simulink model "gm_uz_pmsm_model_9ph_21b_all_double"  (R2021b)
settings: Solver=FixedStepAuto  StartTime=0.0  StopTime=0.8  RelTol=1e-3
PreLoadFcn:
  | uz_pmsm_model_9ph_init_parameter
undefined symbols (not defined in the file or in its folder): a, b, c, friction_coefficient, inertia, k_i_d, k_i_q, k_p_d, k_p_q, Kpd, L_d, L_o1, L_o2, L_q, L_x1, L_x2, L_y1, L_y2, L_zero, polepair, psi_pm, R_1, static_friction_torque, Tnd, ts
libraries: hdlsllib x90, simulink x32, hdlmdlgenlib x17, dspsigops x7, slpidlib x2, spsAlphaBetaZerotodq0Lib x1, pid_lib x1, spsdq0toAlphaBetaZeroLib x1
(part 4 of 6)

== system gm_uz_pmsm_model_9ph_21b_all_double/uz_pmsm_model_9ph/abc_to_dq/abc_to_dq/_adder_MultiplyAdd12 ==
  in0 : Inport  OutDataTypeStr=fixdt(1, 18, 17)  SampleTime=1e-08
  in1 : Inport  Port=2  OutDataTypeStr=fixdt(1, 25, 12)  SampleTime=1e-08
  in2 : Inport  Port=3  OutDataTypeStr=fixdt(1, 25, 12)  SampleTime=1e-08
  globalSchedule : EnablePort  OutDataTypeStr=boolean
  HwModeRegister : Delay  DelayLength=double(1)  InitialCondition=0
  HwModeRegister1 : Delay  DelayLength=double(1)  InitialCondition=0
  HwModeRegister2 : Delay  DelayLength=double(1)  InitialCondition=0
  PipelineRegister : Delay  DelayLength=double(2)  InitialCondition=0
  _adder_MultiplyAdd : hdlsllib/HDL Operations/Multiply-Add  Function=c+(a.*b)  datatype=fixdt(1, 44, 29)  DoSatur=off  FMA=off
      settings: SourceProductBaseCode=SL
  out0 : Outport  OutDataTypeStr=fixdt(1, 44, 29)  SampleTime=1e-08  InitialOutput=0
  wires:
  PipelineRegister/1 -> out0/1
  in0/1 -> HwModeRegister/1
  in1/1 -> HwModeRegister1/1
  in2/1 -> HwModeRegister2/1
  _adder_MultiplyAdd/1 -> PipelineRegister/1
  HwModeRegister/1 -> _adder_MultiplyAdd/1
  HwModeRegister1/1 -> _adder_MultiplyAdd/2
  HwModeRegister2/1 -> _adder_MultiplyAdd/3

== system gm_uz_pmsm_model_9ph_21b_all_double/uz_pmsm_model_9ph/abc_to_dq/abc_to_dq/_adder_MultiplyAdd13 ==
  in0 : Inport  OutDataTypeStr=fixdt(1, 18, 17)  SampleTime=1e-08
  in1 : Inport  Port=2  OutDataTypeStr=fixdt(1, 25, 12)  SampleTime=1e-08
  in2 : Inport  Port=3  OutDataTypeStr=fixdt(1, 25, 12)  SampleTime=1e-08
  globalSchedule : EnablePort  OutDataTypeStr=boolean
  HwModeRegister : Delay  DelayLength=double(1)  InitialCondition=0
  HwModeRegister1 : Delay  DelayLength=double(1)  InitialCondition=0
  HwModeRegister2 : Delay  DelayLength=double(1)  InitialCondition=0
  PipelineRegister : Delay  DelayLength=double(2)  InitialCondition=0
  _adder_MultiplyAdd : hdlsllib/HDL Operations/Multiply-Add  Function=c+(a.*b)  datatype=fixdt(1, 44, 29)  DoSatur=off  FMA=off
      settings: SourceProductBaseCode=SL
  out0 : Outport  OutDataTypeStr=fixdt(1, 44, 29)  SampleTime=1e-08  InitialOutput=0
  wires:
  PipelineRegister/1 -> out0/1
  in0/1 -> HwModeRegister/1
  in1/1 -> HwModeRegister1/1
  in2/1 -> HwModeRegister2/1
  _adder_MultiplyAdd/1 -> PipelineRegister/1
  HwModeRegister/1 -> _adder_MultiplyAdd/1
  HwModeRegister1/1 -> _adder_MultiplyAdd/2
  HwModeRegister2/1 -> _adder_MultiplyAdd/3

== system gm_uz_pmsm_model_9ph_21b_all_double/uz_pmsm_model_9ph/abc_to_dq/abc_to_dq/_adder_MultiplyAdd14 ==
  in0 : Inport  OutDataTypeStr=fixdt(1, 18, 17)  SampleTime=1e-08
  in1 : Inport  Port=2  OutDataTypeStr=fixdt(1, 25, 12)  SampleTime=1e-08
  in2 : Inport  Port=3  OutDataTypeStr=fixdt(1, 25, 12)  SampleTime=1e-08
  globalSchedule : EnablePort  OutDataTypeStr=boolean
  HwModeRegister : Delay  DelayLength=double(1)  InitialCondition=0
  HwModeRegister1 : Delay  DelayLength=double(1)  InitialCondition=0
  HwModeRegister2 : Delay  DelayLength=double(1)  InitialCondition=0
  PipelineRegister : Delay  DelayLength=double(2)  InitialCondition=0
  _adder_MultiplyAdd : hdlsllib/HDL Operations/Multiply-Add  Function=c+(a.*b)  datatype=fixdt(1, 44, 29)  DoSatur=off  FMA=off
      settings: SourceProductBaseCode=SL
  out0 : Outport  OutDataTypeStr=fixdt(1, 44, 29)  SampleTime=1e-08  InitialOutput=0
  wires:
  PipelineRegister/1 -> out0/1
  in0/1 -> HwModeRegister/1
  in1/1 -> HwModeRegister1/1
  in2/1 -> HwModeRegister2/1
  _adder_MultiplyAdd/1 -> PipelineRegister/1
  HwModeRegister/1 -> _adder_MultiplyAdd/1
  HwModeRegister1/1 -> _adder_MultiplyAdd/2
  HwModeRegister2/1 -> _adder_MultiplyAdd/3

== system gm_uz_pmsm_model_9ph_21b_all_double/uz_pmsm_model_9ph/abc_to_dq/abc_to_dq/_adder_MultiplyAdd15 ==
  in0 : Inport  OutDataTypeStr=fixdt(1, 18, 17)  SampleTime=1e-08
  in1 : Inport  Port=2  OutDataTypeStr=fixdt(1, 25, 12)  SampleTime=1e-08
  in2 : Inport  Port=3  OutDataTypeStr=fixdt(1, 25, 12)  SampleTime=1e-08
  globalSchedule : EnablePort  OutDataTypeStr=boolean
  HwModeRegister : Delay  DelayLength=double(1)  InitialCondition=0
  HwModeRegister1 : Delay  DelayLength=double(1)  InitialCondition=0
  HwModeRegister2 : Delay  DelayLength=double(1)  InitialCondition=0
  PipelineRegister : Delay  DelayLength=double(2)  InitialCondition=0
  _adder_MultiplyAdd : hdlsllib/HDL Operations/Multiply-Add  Function=c+(a.*b)  datatype=fixdt(1, 44, 29)  DoSatur=off  FMA=off
      settings: SourceProductBaseCode=SL
  out0 : Outport  OutDataTypeStr=fixdt(1, 44, 29)  SampleTime=1e-08  InitialOutput=0
  wires:
  PipelineRegister/1 -> out0/1
  in0/1 -> HwModeRegister/1
  in1/1 -> HwModeRegister1/1
  in2/1 -> HwModeRegister2/1
  _adder_MultiplyAdd/1 -> PipelineRegister/1
  HwModeRegister/1 -> _adder_MultiplyAdd/1
  HwModeRegister1/1 -> _adder_MultiplyAdd/2
  HwModeRegister2/1 -> _adder_MultiplyAdd/3

== system gm_uz_pmsm_model_9ph_21b_all_double/uz_pmsm_model_9ph/abc_to_dq/abc_to_dq/_adder_MultiplyAdd16 ==
  in0 : Inport  OutDataTypeStr=fixdt(1, 18, 17)  SampleTime=1e-08
  in1 : Inport  Port=2  OutDataTypeStr=fixdt(1, 25, 12)  SampleTime=1e-08
  in2 : Inport  Port=3  OutDataTypeStr=fixdt(1, 25, 12)  SampleTime=1e-08
  globalSchedule : EnablePort  OutDataTypeStr=boolean
  HwModeRegister : Delay  DelayLength=double(1)  InitialCondition=0
  HwModeRegister1 : Delay  DelayLength=double(1)  InitialCondition=0
  HwModeRegister2 : Delay  DelayLength=double(1)  InitialCondition=0
  PipelineRegister : Delay  DelayLength=double(2)  InitialCondition=0
  _adder_MultiplyAdd : hdlsllib/HDL Operations/Multiply-Add  Function=c+(a.*b)  datatype=fixdt(1, 44, 29)  DoSatur=off  FMA=off
      settings: SourceProductBaseCode=SL
  out0 : Outport  OutDataTypeStr=fixdt(1, 44, 29)  SampleTime=1e-08  InitialOutput=0
  wires:
  PipelineRegister/1 -> out0/1
  in0/1 -> HwModeRegister/1
  in1/1 -> HwModeRegister1/1
  in2/1 -> HwModeRegister2/1
  _adder_MultiplyAdd/1 -> PipelineRegister/1
  HwModeRegister/1 -> _adder_MultiplyAdd/1
  HwModeRegister1/1 -> _adder_MultiplyAdd/2
  HwModeRegister2/1 -> _adder_MultiplyAdd/3

== system gm_uz_pmsm_model_9ph_21b_all_double/uz_pmsm_model_9ph/abc_to_dq/abc_to_dq/_adder_MultiplyAdd17 ==
  in0 : Inport  OutDataTypeStr=fixdt(1, 18, 17)  SampleTime=1e-08
  in1 : Inport  Port=2  OutDataTypeStr=fixdt(1, 25, 12)  SampleTime=1e-08
  in2 : Inport  Port=3  OutDataTypeStr=fixdt(1, 25, 12)  SampleTime=1e-08
  globalSchedule : EnablePort  OutDataTypeStr=boolean
  HwModeRegister : Delay  DelayLength=double(1)  InitialCondition=0
  HwModeRegister1 : Delay  DelayLength=double(1)  InitialCondition=0
  HwModeRegister2 : Delay  DelayLength=double(1)  InitialCondition=0
  PipelineRegister : Delay  DelayLength=double(2)  InitialCondition=0
  _adder_MultiplyAdd : hdlsllib/HDL Operations/Multiply-Add  Function=c+(a.*b)  datatype=fixdt(1, 44, 29)  DoSatur=off  FMA=off
      settings: SourceProductBaseCode=SL
  out0 : Outport  OutDataTypeStr=fixdt(1, 44, 29)  SampleTime=1e-08  InitialOutput=0
  wires:
  PipelineRegister/1 -> out0/1
  in0/1 -> HwModeRegister/1
  in1/1 -> HwModeRegister1/1
  in2/1 -> HwModeRegister2/1
  _adder_MultiplyAdd/1 -> PipelineRegister/1
  HwModeRegister/1 -> _adder_MultiplyAdd/1
  HwModeRegister1/1 -> _adder_MultiplyAdd/2
  HwModeRegister2/1 -> _adder_MultiplyAdd/3

== system gm_uz_pmsm_model_9ph_21b_all_double/uz_pmsm_model_9ph/abc_to_dq/abc_to_dq/_adder_MultiplyAdd18 ==
  in0 : Inport  OutDataTypeStr=fixdt(1, 18, 17)  SampleTime=1e-08
  in1 : Inport  Port=2  OutDataTypeStr=fixdt(1, 25, 12)  SampleTime=1e-08
  in2 : Inport  Port=3  OutDataTypeStr=fixdt(1, 25, 12)  SampleTime=1e-08
  globalSchedule : EnablePort  OutDataTypeStr=boolean
  HwModeRegister : Delay  DelayLength=double(1)  InitialCondition=0
  HwModeRegister1 : Delay  DelayLength=double(1)  InitialCondition=0
  HwModeRegister2 : Delay  DelayLength=double(1)  InitialCondition=0
  PipelineRegister : Delay  DelayLength=double(2)  InitialCondition=0
  _adder_MultiplyAdd : hdlsllib/HDL Operations/Multiply-Add  Function=c+(a.*b)  datatype=fixdt(1, 44, 29)  DoSatur=off  FMA=off
      settings: SourceProductBaseCode=SL
  out0 : Outport  OutDataTypeStr=fixdt(1, 44, 29)  SampleTime=1e-08  InitialOutput=0
  wires:
  PipelineRegister/1 -> out0/1
  in0/1 -> HwModeRegister/1
  in1/1 -> HwModeRegister1/1
  in2/1 -> HwModeRegister2/1
  _adder_MultiplyAdd/1 -> PipelineRegister/1
  HwModeRegister/1 -> _adder_MultiplyAdd/1
  HwModeRegister1/1 -> _adder_MultiplyAdd/2
  HwModeRegister2/1 -> _adder_MultiplyAdd/3

== system gm_uz_pmsm_model_9ph_21b_all_double/uz_pmsm_model_9ph/abc_to_dq/abc_to_dq/_adder_MultiplyAdd19 ==
  in0 : Inport  OutDataTypeStr=fixdt(1, 18, 17)  SampleTime=1e-08
  in1 : Inport  Port=2  OutDataTypeStr=fixdt(1, 25, 12)  SampleTime=1e-08
  in2 : Inport  Port=3  OutDataTypeStr=fixdt(1, 25, 12)  SampleTime=1e-08
  globalSchedule : EnablePort  OutDataTypeStr=boolean
  HwModeRegister : Delay  DelayLength=double(1)  InitialCondition=0
  HwModeRegister1 : Delay  DelayLength=double(1)  InitialCondition=0
  HwModeRegister2 : Delay  DelayLength=double(1)  InitialCondition=0
  PipelineRegister : Delay  DelayLength=double(2)  InitialCondition=0
  _adder_MultiplyAdd : hdlsllib/HDL Operations/Multiply-Add  Function=c+(a.*b)  datatype=fixdt(1, 44, 29)  DoSatur=off  FMA=off
      settings: SourceProductBaseCode=SL
  out0 : Outport  OutDataTypeStr=fixdt(1, 44, 29)  SampleTime=1e-08  InitialOutput=0
  wires:
  PipelineRegister/1 -> out0/1
  in0/1 -> HwModeRegister/1
  in1/1 -> HwModeRegister1/1
  in2/1 -> HwModeRegister2/1
  _adder_MultiplyAdd/1 -> PipelineRegister/1
  HwModeRegister/1 -> _adder_MultiplyAdd/1
  HwModeRegister1/1 -> _adder_MultiplyAdd/2
  HwModeRegister2/1 -> _adder_MultiplyAdd/3

== system gm_uz_pmsm_model_9ph_21b_all_double/uz_pmsm_model_9ph/abc_to_dq/abc_to_dq/_adder_MultiplyAdd2 ==
  in0 : Inport  OutDataTypeStr=fixdt(1, 18, 17)  SampleTime=1e-08
  in1 : Inport  Port=2  OutDataTypeStr=fixdt(1, 25, 12)  SampleTime=1e-08
  in2 : Inport  Port=3  OutDataTypeStr=fixdt(1, 25, 12)  SampleTime=1e-08
  globalSchedule : EnablePort  OutDataTypeStr=boolean
  HwModeRegister : Delay  DelayLength=double(1)  InitialCondition=0
  HwModeRegister1 : Delay  DelayLength=double(1)  InitialCondition=0
  HwModeRegister2 : Delay  DelayLength=double(1)  InitialCondition=0
  PipelineRegister : Delay  DelayLength=double(2)  InitialCondition=0
  _adder_MultiplyAdd : hdlsllib/HDL Operations/Multiply-Add  Function=c+(a.*b)  datatype=fixdt(1, 44, 29)  DoSatur=off  FMA=off
      settings: SourceProductBaseCode=SL
  out0 : Outport  OutDataTypeStr=fixdt(1, 44, 29)  SampleTime=1e-08  InitialOutput=0
  wires:
  PipelineRegister/1 -> out0/1
  in0/1 -> HwModeRegister/1
  in1/1 -> HwModeRegister1/1
  in2/1 -> HwModeRegister2/1
  _adder_MultiplyAdd/1 -> PipelineRegister/1
  HwModeRegister/1 -> _adder_MultiplyAdd/1
  HwModeRegister1/1 -> _adder_MultiplyAdd/2
  HwModeRegister2/1 -> _adder_MultiplyAdd/3

== system gm_uz_pmsm_model_9ph_21b_all_double/uz_pmsm_model_9ph/abc_to_dq/abc_to_dq/_adder_MultiplyAdd20 ==
  in0 : Inport  OutDataTypeStr=fixdt(1, 18, 17)  SampleTime=1e-08
  in1 : Inport  Port=2  OutDataTypeStr=fixdt(1, 25, 12)  SampleTime=1e-08
  in2 : Inport  Port=3  OutDataTypeStr=fixdt(1, 25, 12)  SampleTime=1e-08
  globalSchedule : EnablePort  OutDataTypeStr=boolean
  HwModeRegister : Delay  DelayLength=double(1)  InitialCondition=0
  HwModeRegister1 : Delay  DelayLength=double(1)  InitialCondition=0
  HwModeRegister2 : Delay  DelayLength=double(1)  InitialCondition=0
  PipelineRegister : Delay  DelayLength=double(2)  InitialCondition=0
  _adder_MultiplyAdd : hdlsllib/HDL Operations/Multiply-Add  Function=c+(a.*b)  datatype=fixdt(1, 44, 29)  DoSatur=off  FMA=off
      settings: SourceProductBaseCode=SL
  out0 : Outport  OutDataTypeStr=fixdt(1, 44, 29)  SampleTime=1e-08  InitialOutput=0
  wires:
  PipelineRegister/1 -> out0/1
  in0/1 -> HwModeRegister/1
  in1/1 -> HwModeRegister1/1
  in2/1 -> HwModeRegister2/1
  _adder_MultiplyAdd/1 -> PipelineRegister/1
  HwModeRegister/1 -> _adder_MultiplyAdd/1
  HwModeRegister1/1 -> _adder_MultiplyAdd/2
  HwModeRegister2/1 -> _adder_MultiplyAdd/3

== system gm_uz_pmsm_model_9ph_21b_all_double/uz_pmsm_model_9ph/abc_to_dq/abc_to_dq/_adder_MultiplyAdd21 ==
  in0 : Inport  OutDataTypeStr=fixdt(1, 18, 17)  SampleTime=1e-08
  in1 : Inport  Port=2  OutDataTypeStr=fixdt(1, 25, 12)  SampleTime=1e-08
  in2 : Inport  Port=3  OutDataTypeStr=fixdt(1, 25, 12)  SampleTime=1e-08
  globalSchedule : EnablePort  OutDataTypeStr=boolean
  HwModeRegister : Delay  DelayLength=double(1)  InitialCondition=0
  HwModeRegister1 : Delay  DelayLength=double(1)  InitialCondition=0
  HwModeRegister2 : Delay  DelayLength=double(1)  InitialCondition=0
  PipelineRegister : Delay  DelayLength=double(2)  InitialCondition=0
  _adder_MultiplyAdd : hdlsllib/HDL Operations/Multiply-Add  Function=c+(a.*b)  datatype=fixdt(1, 44, 29)  DoSatur=off  FMA=off
      settings: SourceProductBaseCode=SL
  out0 : Outport  OutDataTypeStr=fixdt(1, 44, 29)  SampleTime=1e-08  InitialOutput=0
  wires:
  PipelineRegister/1 -> out0/1
  in0/1 -> HwModeRegister/1
  in1/1 -> HwModeRegister1/1
  in2/1 -> HwModeRegister2/1
  _adder_MultiplyAdd/1 -> PipelineRegister/1
  HwModeRegister/1 -> _adder_MultiplyAdd/1
  HwModeRegister1/1 -> _adder_MultiplyAdd/2
  HwModeRegister2/1 -> _adder_MultiplyAdd/3

== system gm_uz_pmsm_model_9ph_21b_all_double/uz_pmsm_model_9ph/abc_to_dq/abc_to_dq/_adder_MultiplyAdd22 ==
  in0 : Inport  OutDataTypeStr=fixdt(1, 18, 17)  SampleTime=1e-08
  in1 : Inport  Port=2  OutDataTypeStr=fixdt(1, 25, 12)  SampleTime=1e-08
  in2 : Inport  Port=3  OutDataTypeStr=fixdt(1, 25, 12)  SampleTime=1e-08
  globalSchedule : EnablePort  OutDataTypeStr=boolean
  HwModeRegister : Delay  DelayLength=double(1)  InitialCondition=0
  HwModeRegister1 : Delay  DelayLength=double(1)  InitialCondition=0
  HwModeRegister2 : Delay  DelayLength=double(1)  InitialCondition=0
  PipelineRegister : Delay  DelayLength=double(2)  InitialCondition=0
  _adder_MultiplyAdd : hdlsllib/HDL Operations/Multiply-Add  Function=c+(a.*b)  datatype=fixdt(1, 44, 29)  DoSatur=off  FMA=off
      settings: SourceProductBaseCode=SL
  out0 : Outport  OutDataTypeStr=fixdt(1, 44, 29)  SampleTime=1e-08  InitialOutput=0
  wires:
  PipelineRegister/1 -> out0/1
  in0/1 -> HwModeRegister/1
  in1/1 -> HwModeRegister1/1
  in2/1 -> HwModeRegister2/1
  _adder_MultiplyAdd/1 -> PipelineRegister/1
  HwModeRegister/1 -> _adder_MultiplyAdd/1
  HwModeRegister1/1 -> _adder_MultiplyAdd/2
  HwModeRegister2/1 -> _adder_MultiplyAdd/3

== system gm_uz_pmsm_model_9ph_21b_all_double/uz_pmsm_model_9ph/abc_to_dq/abc_to_dq/_adder_MultiplyAdd23 ==
  in0 : Inport  OutDataTypeStr=fixdt(1, 18, 17)  SampleTime=1e-08
  in1 : Inport  Port=2  OutDataTypeStr=fixdt(1, 25, 12)  SampleTime=1e-08
  in2 : Inport  Port=3  OutDataTypeStr=fixdt(1, 25, 12)  SampleTime=1e-08
  globalSchedule : EnablePort  OutDataTypeStr=boolean
  HwModeRegister : Delay  DelayLength=double(1)  InitialCondition=0
  HwModeRegister1 : Delay  DelayLength=double(1)  InitialCondition=0
  HwModeRegister2 : Delay  DelayLength=double(1)  InitialCondition=0
  PipelineRegister : Delay  DelayLength=double(2)  InitialCondition=0
  _adder_MultiplyAdd : hdlsllib/HDL Operations/Multiply-Add  Function=c+(a.*b)  datatype=fixdt(1, 44, 29)  DoSatur=off  FMA=off
      settings: SourceProductBaseCode=SL
  out0 : Outport  OutDataTypeStr=fixdt(1, 44, 29)  SampleTime=1e-08  InitialOutput=0
  wires:
  PipelineRegister/1 -> out0/1
  in0/1 -> HwModeRegister/1
  in1/1 -> HwModeRegister1/1
  in2/1 -> HwModeRegister2/1
  _adder_MultiplyAdd/1 -> PipelineRegister/1
  HwModeRegister/1 -> _adder_MultiplyAdd/1
  HwModeRegister1/1 -> _adder_MultiplyAdd/2
  HwModeRegister2/1 -> _adder_MultiplyAdd/3

== system gm_uz_pmsm_model_9ph_21b_all_double/uz_pmsm_model_9ph/abc_to_dq/abc_to_dq/_adder_MultiplyAdd24 ==
  in0 : Inport  OutDataTypeStr=fixdt(1, 18, 17)  SampleTime=1e-08
  in1 : Inport  Port=2  OutDataTypeStr=fixdt(1, 25, 12)  SampleTime=1e-08
  in2 : Inport  Port=3  OutDataTypeStr=fixdt(1, 25, 12)  SampleTime=1e-08
  globalSchedule : EnablePort  OutDataTypeStr=boolean
  HwModeRegister : Delay  DelayLength=double(1)  InitialCondition=0
  HwModeRegister1 : Delay  DelayLength=double(1)  InitialCondition=0
  HwModeRegister2 : Delay  DelayLength=double(1)  InitialCondition=0
  PipelineRegister : Delay  DelayLength=double(2)  InitialCondition=0
  _adder_MultiplyAdd : hdlsllib/HDL Operations/Multiply-Add  Function=c+(a.*b)  datatype=fixdt(1, 44, 29)  DoSatur=off  FMA=off
      settings: SourceProductBaseCode=SL
  out0 : Outport  OutDataTypeStr=fixdt(1, 44, 29)  SampleTime=1e-08  InitialOutput=0
  wires:
  PipelineRegister/1 -> out0/1
  in0/1 -> HwModeRegister/1
  in1/1 -> HwModeRegister1/1
  in2/1 -> HwModeRegister2/1
  _adder_MultiplyAdd/1 -> PipelineRegister/1
  HwModeRegister/1 -> _adder_MultiplyAdd/1
  HwModeRegister1/1 -> _adder_MultiplyAdd/2
  HwModeRegister2/1 -> _adder_MultiplyAdd/3

== system gm_uz_pmsm_model_9ph_21b_all_double/uz_pmsm_model_9ph/abc_to_dq/abc_to_dq/_adder_MultiplyAdd25 ==
  in0 : Inport  OutDataTypeStr=fixdt(1, 18, 17)  SampleTime=1e-08
  in1 : Inport  Port=2  OutDataTypeStr=fixdt(1, 25, 12)  SampleTime=1e-08
  in2 : Inport  Port=3  OutDataTypeStr=fixdt(1, 25, 12)  SampleTime=1e-08
  globalSchedule : EnablePort  OutDataTypeStr=boolean
  HwModeRegister : Delay  DelayLength=double(1)  InitialCondition=0
  HwModeRegister1 : Delay  DelayLength=double(1)  InitialCondition=0
  HwModeRegister2 : Delay  DelayLength=double(1)  InitialCondition=0
  PipelineRegister : Delay  DelayLength=double(2)  InitialCondition=0
  _adder_MultiplyAdd : hdlsllib/HDL Operations/Multiply-Add  Function=c+(a.*b)  datatype=fixdt(1, 44, 29)  DoSatur=off  FMA=off
      settings: SourceProductBaseCode=SL
  out0 : Outport  OutDataTypeStr=fixdt(1, 44, 29)  SampleTime=1e-08  InitialOutput=0
  wires:
  PipelineRegister/1 -> out0/1
  in0/1 -> HwModeRegister/1
  in1/1 -> HwModeRegister1/1
  in2/1 -> HwModeRegister2/1
  _adder_MultiplyAdd/1 -> PipelineRegister/1
  HwModeRegister/1 -> _adder_MultiplyAdd/1
  HwModeRegister1/1 -> _adder_MultiplyAdd/2
  HwModeRegister2/1 -> _adder_MultiplyAdd/3

== system gm_uz_pmsm_model_9ph_21b_all_double/uz_pmsm_model_9ph/abc_to_dq/abc_to_dq/_adder_MultiplyAdd26 ==
  in0 : Inport  OutDataTypeStr=fixdt(1, 18, 17)  SampleTime=1e-08
  in1 : Inport  Port=2  OutDataTypeStr=fixdt(1, 25, 12)  SampleTime=1e-08
  in2 : Inport  Port=3  OutDataTypeStr=fixdt(1, 25, 12)  SampleTime=1e-08
  globalSchedule : EnablePort  OutDataTypeStr=boolean
  HwModeRegister : Delay  DelayLength=double(1)  InitialCondition=0
  HwModeRegister1 : Delay  DelayLength=double(1)  InitialCondition=0
  HwModeRegister2 : Delay  DelayLength=double(1)  InitialCondition=0
  PipelineRegister : Delay  DelayLength=double(2)  InitialCondition=0
  _adder_MultiplyAdd : hdlsllib/HDL Operations/Multiply-Add  Function=c+(a.*b)  datatype=fixdt(1, 44, 29)  DoSatur=off  FMA=off
      settings: SourceProductBaseCode=SL
  out0 : Outport  OutDataTypeStr=fixdt(1, 44, 29)  SampleTime=1e-08  InitialOutput=0
  wires:
  PipelineRegister/1 -> out0/1
  in0/1 -> HwModeRegister/1
  in1/1 -> HwModeRegister1/1
  in2/1 -> HwModeRegister2/1
  _adder_MultiplyAdd/1 -> PipelineRegister/1
  HwModeRegister/1 -> _adder_MultiplyAdd/1
  HwModeRegister1/1 -> _adder_MultiplyAdd/2
  HwModeRegister2/1 -> _adder_MultiplyAdd/3

== system gm_uz_pmsm_model_9ph_21b_all_double/uz_pmsm_model_9ph/abc_to_dq/abc_to_dq/_adder_MultiplyAdd27 ==
  in0 : Inport  OutDataTypeStr=fixdt(1, 18, 17)  SampleTime=1e-08
  in1 : Inport  Port=2  OutDataTypeStr=fixdt(1, 25, 12)  SampleTime=1e-08
  in2 : Inport  Port=3  OutDataTypeStr=fixdt(1, 25, 12)  SampleTime=1e-08
  globalSchedule : EnablePort  OutDataTypeStr=boolean
  HwModeRegister : Delay  DelayLength=double(1)  InitialCondition=0
  HwModeRegister1 : Delay  DelayLength=double(1)  InitialCondition=0
  HwModeRegister2 : Delay  DelayLength=double(1)  InitialCondition=0
  PipelineRegister : Delay  DelayLength=double(2)  InitialCondition=0
  _adder_MultiplyAdd : hdlsllib/HDL Operations/Multiply-Add  Function=c+(a.*b)  datatype=fixdt(1, 44, 29)  DoSatur=off  FMA=off
      settings: SourceProductBaseCode=SL
  out0 : Outport  OutDataTypeStr=fixdt(1, 44, 29)  SampleTime=1e-08  InitialOutput=0
  wires:
  PipelineRegister/1 -> out0/1
  in0/1 -> HwModeRegister/1
  in1/1 -> HwModeRegister1/1
  in2/1 -> HwModeRegister2/1
  _adder_MultiplyAdd/1 -> PipelineRegister/1
  HwModeRegister/1 -> _adder_MultiplyAdd/1
  HwModeRegister1/1 -> _adder_MultiplyAdd/2
  HwModeRegister2/1 -> _adder_MultiplyAdd/3

== system gm_uz_pmsm_model_9ph_21b_all_double/uz_pmsm_model_9ph/abc_to_dq/abc_to_dq/_adder_MultiplyAdd28 ==
  in0 : Inport  OutDataTypeStr=fixdt(1, 18, 17)  SampleTime=1e-08
  in1 : Inport  Port=2  OutDataTypeStr=fixdt(1, 25, 12)  SampleTime=1e-08
  in2 : Inport  Port=3  OutDataTypeStr=fixdt(1, 25, 12)  SampleTime=1e-08
  globalSchedule : EnablePort  OutDataTypeStr=boolean
  HwModeRegister : Delay  DelayLength=double(1)  InitialCondition=0
  HwModeRegister1 : Delay  DelayLength=double(1)  InitialCondition=0
  HwModeRegister2 : Delay  DelayLength=double(1)  InitialCondition=0
  PipelineRegister : Delay  DelayLength=double(2)  InitialCondition=0
  _adder_MultiplyAdd : hdlsllib/HDL Operations/Multiply-Add  Function=c+(a.*b)  datatype=fixdt(1, 44, 29)  DoSatur=off  FMA=off
      settings: SourceProductBaseCode=SL
  out0 : Outport  OutDataTypeStr=fixdt(1, 44, 29)  SampleTime=1e-08  InitialOutput=0
  wires:
  PipelineRegister/1 -> out0/1
  in0/1 -> HwModeRegister/1
  in1/1 -> HwModeRegister1/1
  in2/1 -> HwModeRegister2/1
  _adder_MultiplyAdd/1 -> PipelineRegister/1
  HwModeRegister/1 -> _adder_MultiplyAdd/1
  HwModeRegister1/1 -> _adder_MultiplyAdd/2
  HwModeRegister2/1 -> _adder_MultiplyAdd/3

== system gm_uz_pmsm_model_9ph_21b_all_double/uz_pmsm_model_9ph/abc_to_dq/abc_to_dq/_adder_MultiplyAdd29 ==
  in0 : Inport  OutDataTypeStr=fixdt(1, 18, 17)  SampleTime=1e-08
  in1 : Inport  Port=2  OutDataTypeStr=fixdt(1, 25, 12)  SampleTime=1e-08
  in2 : Inport  Port=3  OutDataTypeStr=fixdt(1, 25, 12)  SampleTime=1e-08
  globalSchedule : EnablePort  OutDataTypeStr=boolean
  HwModeRegister : Delay  DelayLength=double(1)  InitialCondition=0
  HwModeRegister1 : Delay  DelayLength=double(1)  InitialCondition=0
  HwModeRegister2 : Delay  DelayLength=double(1)  InitialCondition=0
  PipelineRegister : Delay  DelayLength=double(2)  InitialCondition=0
  _adder_MultiplyAdd : hdlsllib/HDL Operations/Multiply-Add  Function=c+(a.*b)  datatype=fixdt(1, 44, 29)  DoSatur=off  FMA=off
      settings: SourceProductBaseCode=SL
  out0 : Outport  OutDataTypeStr=fixdt(1, 44, 29)  SampleTime=1e-08  InitialOutput=0
  wires:
  PipelineRegister/1 -> out0/1
  in0/1 -> HwModeRegister/1
  in1/1 -> HwModeRegister1/1
  in2/1 -> HwModeRegister2/1
  _adder_MultiplyAdd/1 -> PipelineRegister/1
  HwModeRegister/1 -> _adder_MultiplyAdd/1
  HwModeRegister1/1 -> _adder_MultiplyAdd/2
  HwModeRegister2/1 -> _adder_MultiplyAdd/3

== system gm_uz_pmsm_model_9ph_21b_all_double/uz_pmsm_model_9ph/abc_to_dq/abc_to_dq/_adder_MultiplyAdd3 ==
  in0 : Inport  OutDataTypeStr=fixdt(1, 18, 17)  SampleTime=1e-08
  in1 : Inport  Port=2  OutDataTypeStr=fixdt(1, 25, 12)  SampleTime=1e-08
  in2 : Inport  Port=3  OutDataTypeStr=fixdt(1, 25, 12)  SampleTime=1e-08
  globalSchedule : EnablePort  OutDataTypeStr=boolean
  HwModeRegister : Delay  DelayLength=double(1)  InitialCondition=0
  HwModeRegister1 : Delay  DelayLength=double(1)  InitialCondition=0
  HwModeRegister2 : Delay  DelayLength=double(1)  InitialCondition=0
  PipelineRegister : Delay  DelayLength=double(2)  InitialCondition=0
  _adder_MultiplyAdd : hdlsllib/HDL Operations/Multiply-Add  Function=c+(a.*b)  datatype=fixdt(1, 44, 29)  DoSatur=off  FMA=off
      settings: SourceProductBaseCode=SL
  out0 : Outport  OutDataTypeStr=fixdt(1, 44, 29)  SampleTime=1e-08  InitialOutput=0
  wires:
  PipelineRegister/1 -> out0/1
  in0/1 -> HwModeRegister/1
  in1/1 -> HwModeRegister1/1
  in2/1 -> HwModeRegister2/1
  _adder_MultiplyAdd/1 -> PipelineRegister/1
  HwModeRegister/1 -> _adder_MultiplyAdd/1
  HwModeRegister1/1 -> _adder_MultiplyAdd/2
  HwModeRegister2/1 -> _adder_MultiplyAdd/3

== system gm_uz_pmsm_model_9ph_21b_all_double/uz_pmsm_model_9ph/abc_to_dq/abc_to_dq/_adder_MultiplyAdd30 ==
  in0 : Inport  OutDataTypeStr=fixdt(1, 18, 17)  SampleTime=1e-08
  in1 : Inport  Port=2  OutDataTypeStr=fixdt(1, 25, 12)  SampleTime=1e-08
  in2 : Inport  Port=3  OutDataTypeStr=fixdt(1, 25, 12)  SampleTime=1e-08
  globalSchedule : EnablePort  OutDataTypeStr=boolean
  HwModeRegister : Delay  DelayLength=double(1)  InitialCondition=0
  HwModeRegister1 : Delay  DelayLength=double(1)  InitialCondition=0
  HwModeRegister2 : Delay  DelayLength=double(1)  InitialCondition=0
  PipelineRegister : Delay  DelayLength=double(2)  InitialCondition=0
  _adder_MultiplyAdd : hdlsllib/HDL Operations/Multiply-Add  Function=c+(a.*b)  datatype=fixdt(1, 44, 29)  DoSatur=off  FMA=off
      settings: SourceProductBaseCode=SL
  out0 : Outport  OutDataTypeStr=fixdt(1, 44, 29)  SampleTime=1e-08  InitialOutput=0
  wires:
  PipelineRegister/1 -> out0/1
  in0/1 -> HwModeRegister/1
  in1/1 -> HwModeRegister1/1
  in2/1 -> HwModeRegister2/1
  _adder_MultiplyAdd/1 -> PipelineRegister/1
  HwModeRegister/1 -> _adder_MultiplyAdd/1
  HwModeRegister1/1 -> _adder_MultiplyAdd/2
  HwModeRegister2/1 -> _adder_MultiplyAdd/3

== system gm_uz_pmsm_model_9ph_21b_all_double/uz_pmsm_model_9ph/abc_to_dq/abc_to_dq/_adder_MultiplyAdd31 ==
  in0 : Inport  OutDataTypeStr=fixdt(1, 18, 17)  SampleTime=1e-08
  in1 : Inport  Port=2  OutDataTypeStr=fixdt(1, 25, 12)  SampleTime=1e-08
  in2 : Inport  Port=3  OutDataTypeStr=fixdt(1, 25, 12)  SampleTime=1e-08
  globalSchedule : EnablePort  OutDataTypeStr=boolean
  HwModeRegister : Delay  DelayLength=double(1)  InitialCondition=0
  HwModeRegister1 : Delay  DelayLength=double(1)  InitialCondition=0
  HwModeRegister2 : Delay  DelayLength=double(1)  InitialCondition=0
  PipelineRegister : Delay  DelayLength=double(2)  InitialCondition=0
  _adder_MultiplyAdd : hdlsllib/HDL Operations/Multiply-Add  Function=c+(a.*b)  datatype=fixdt(1, 44, 29)  DoSatur=off  FMA=off
      settings: SourceProductBaseCode=SL
  out0 : Outport  OutDataTypeStr=fixdt(1, 44, 29)  SampleTime=1e-08  InitialOutput=0
  wires:
  PipelineRegister/1 -> out0/1
  in0/1 -> HwModeRegister/1
  in1/1 -> HwModeRegister1/1
  in2/1 -> HwModeRegister2/1
  _adder_MultiplyAdd/1 -> PipelineRegister/1
  HwModeRegister/1 -> _adder_MultiplyAdd/1
  HwModeRegister1/1 -> _adder_MultiplyAdd/2
  HwModeRegister2/1 -> _adder_MultiplyAdd/3

== system gm_uz_pmsm_model_9ph_21b_all_double/uz_pmsm_model_9ph/abc_to_dq/abc_to_dq/_adder_MultiplyAdd32 ==
  in0 : Inport  OutDataTypeStr=fixdt(1, 18, 17)  SampleTime=1e-08
  in1 : Inport  Port=2  OutDataTypeStr=fixdt(1, 25, 12)  SampleTime=1e-08
  in2 : Inport  Port=3  OutDataTypeStr=fixdt(1, 25, 12)  SampleTime=1e-08
  globalSchedule : EnablePort  OutDataTypeStr=boolean
  HwModeRegister : Delay  DelayLength=double(1)  InitialCondition=0
  HwModeRegister1 : Delay  DelayLength=double(1)  InitialCondition=0
  HwModeRegister2 : Delay  DelayLength=double(1)  InitialCondition=0
  PipelineRegister : Delay  DelayLength=double(2)  InitialCondition=0
  _adder_MultiplyAdd : hdlsllib/HDL Operations/Multiply-Add  Function=c+(a.*b)  datatype=fixdt(1, 44, 29)  DoSatur=off  FMA=off
      settings: SourceProductBaseCode=SL
  out0 : Outport  OutDataTypeStr=fixdt(1, 44, 29)  SampleTime=1e-08  InitialOutput=0
  wires:
  PipelineRegister/1 -> out0/1
  in0/1 -> HwModeRegister/1
  in1/1 -> HwModeRegister1/1
  in2/1 -> HwModeRegister2/1
  _adder_MultiplyAdd/1 -> PipelineRegister/1
  HwModeRegister/1 -> _adder_MultiplyAdd/1
  HwModeRegister1/1 -> _adder_MultiplyAdd/2
  HwModeRegister2/1 -> _adder_MultiplyAdd/3

== system gm_uz_pmsm_model_9ph_21b_all_double/uz_pmsm_model_9ph/abc_to_dq/abc_to_dq/_adder_MultiplyAdd33 ==
  in0 : Inport  OutDataTypeStr=fixdt(1, 18, 17)  SampleTime=1e-08
  in1 : Inport  Port=2  OutDataTypeStr=fixdt(1, 25, 12)  SampleTime=1e-08
  in2 : Inport  Port=3  OutDataTypeStr=fixdt(1, 25, 12)  SampleTime=1e-08
  globalSchedule : EnablePort  OutDataTypeStr=boolean
  HwModeRegister : Delay  DelayLength=double(1)  InitialCondition=0
  HwModeRegister1 : Delay  DelayLength=double(1)  InitialCondition=0
  HwModeRegister2 : Delay  DelayLength=double(1)  InitialCondition=0
  PipelineRegister : Delay  DelayLength=double(2)  InitialCondition=0
  _adder_MultiplyAdd : hdlsllib/HDL Operations/Multiply-Add  Function=c+(a.*b)  datatype=fixdt(1, 44, 29)  DoSatur=off  FMA=off
      settings: SourceProductBaseCode=SL
  out0 : Outport  OutDataTypeStr=fixdt(1, 44, 29)  SampleTime=1e-08  InitialOutput=0
  wires:
  PipelineRegister/1 -> out0/1
  in0/1 -> HwModeRegister/1
  in1/1 -> HwModeRegister1/1
  in2/1 -> HwModeRegister2/1
  _adder_MultiplyAdd/1 -> PipelineRegister/1
  HwModeRegister/1 -> _adder_MultiplyAdd/1
  HwModeRegister1/1 -> _adder_MultiplyAdd/2
  HwModeRegister2/1 -> _adder_MultiplyAdd/3

== system gm_uz_pmsm_model_9ph_21b_all_double/uz_pmsm_model_9ph/abc_to_dq/abc_to_dq/_adder_MultiplyAdd34 ==
  in0 : Inport  OutDataTypeStr=fixdt(1, 18, 17)  SampleTime=1e-08
  in1 : Inport  Port=2  OutDataTypeStr=fixdt(1, 25, 12)  SampleTime=1e-08
  in2 : Inport  Port=3  OutDataTypeStr=fixdt(1, 25, 12)  SampleTime=1e-08
  globalSchedule : EnablePort  OutDataTypeStr=boolean
  HwModeRegister : Delay  DelayLength=double(1)  InitialCondition=0
  HwModeRegister1 : Delay  DelayLength=double(1)  InitialCondition=0
  HwModeRegister2 : Delay  DelayLength=double(1)  InitialCondition=0
  PipelineRegister : Delay  DelayLength=double(2)  InitialCondition=0
  _adder_MultiplyAdd : hdlsllib/HDL Operations/Multiply-Add  Function=c+(a.*b)  datatype=fixdt(1, 44, 29)  DoSatur=off  FMA=off
      settings: SourceProductBaseCode=SL
  out0 : Outport  OutDataTypeStr=fixdt(1, 44, 29)  SampleTime=1e-08  InitialOutput=0
  wires:
  PipelineRegister/1 -> out0/1
  in0/1 -> HwModeRegister/1
  in1/1 -> HwModeRegister1/1
  in2/1 -> HwModeRegister2/1
  _adder_MultiplyAdd/1 -> PipelineRegister/1
  HwModeRegister/1 -> _adder_MultiplyAdd/1
  HwModeRegister1/1 -> _adder_MultiplyAdd/2
  HwModeRegister2/1 -> _adder_MultiplyAdd/3

== system gm_uz_pmsm_model_9ph_21b_all_double/uz_pmsm_model_9ph/abc_to_dq/abc_to_dq/_adder_MultiplyAdd35 ==
  in0 : Inport  OutDataTypeStr=fixdt(1, 18, 17)  SampleTime=1e-08
  in1 : Inport  Port=2  OutDataTypeStr=fixdt(1, 25, 12)  SampleTime=1e-08
  in2 : Inport  Port=3  OutDataTypeStr=fixdt(1, 25, 12)  SampleTime=1e-08
  globalSchedule : EnablePort  OutDataTypeStr=boolean
  HwModeRegister : Delay  DelayLength=double(1)  InitialCondition=0
  HwModeRegister1 : Delay  DelayLength=double(1)  InitialCondition=0
  HwModeRegister2 : Delay  DelayLength=double(1)  InitialCondition=0
  PipelineRegister : Delay  DelayLength=double(2)  InitialCondition=0
  _adder_MultiplyAdd : hdlsllib/HDL Operations/Multiply-Add  Function=c+(a.*b)  datatype=fixdt(1, 44, 29)  DoSatur=off  FMA=off
      settings: SourceProductBaseCode=SL
  out0 : Outport  OutDataTypeStr=fixdt(1, 44, 29)  SampleTime=1e-08  InitialOutput=0
  wires:
  PipelineRegister/1 -> out0/1
  in0/1 -> HwModeRegister/1
  in1/1 -> HwModeRegister1/1
  in2/1 -> HwModeRegister2/1
  _adder_MultiplyAdd/1 -> PipelineRegister/1
  HwModeRegister/1 -> _adder_MultiplyAdd/1
  HwModeRegister1/1 -> _adder_MultiplyAdd/2
  HwModeRegister2/1 -> _adder_MultiplyAdd/3

== system gm_uz_pmsm_model_9ph_21b_all_double/uz_pmsm_model_9ph/abc_to_dq/abc_to_dq/_adder_MultiplyAdd36 ==
  in0 : Inport  OutDataTypeStr=fixdt(1, 18, 17)  SampleTime=1e-08
  in1 : Inport  Port=2  OutDataTypeStr=fixdt(1, 25, 12)  SampleTime=1e-08
  in2 : Inport  Port=3  OutDataTypeStr=fixdt(1, 25, 12)  SampleTime=1e-08
  globalSchedule : EnablePort  OutDataTypeStr=boolean
  HwModeRegister : Delay  DelayLength=double(1)  InitialCondition=0
  HwModeRegister1 : Delay  DelayLength=double(1)  InitialCondition=0
  HwModeRegister2 : Delay  DelayLength=double(1)  InitialCondition=0
  PipelineRegister : Delay  DelayLength=double(2)  InitialCondition=0
  _adder_MultiplyAdd : hdlsllib/HDL Operations/Multiply-Add  Function=c+(a.*b)  datatype=fixdt(1, 44, 29)  DoSatur=off  FMA=off
      settings: SourceProductBaseCode=SL
  out0 : Outport  OutDataTypeStr=fixdt(1, 44, 29)  SampleTime=1e-08  InitialOutput=0
  wires:
  PipelineRegister/1 -> out0/1
  in0/1 -> HwModeRegister/1
  in1/1 -> HwModeRegister1/1
  in2/1 -> HwModeRegister2/1
  _adder_MultiplyAdd/1 -> PipelineRegister/1
  HwModeRegister/1 -> _adder_MultiplyAdd/1
  HwModeRegister1/1 -> _adder_MultiplyAdd/2
  HwModeRegister2/1 -> _adder_MultiplyAdd/3

== system gm_uz_pmsm_model_9ph_21b_all_double/uz_pmsm_model_9ph/abc_to_dq/abc_to_dq/_adder_MultiplyAdd37 ==
  in0 : Inport  OutDataTypeStr=fixdt(1, 18, 17)  SampleTime=1e-08
  in1 : Inport  Port=2  OutDataTypeStr=fixdt(1, 25, 12)  SampleTime=1e-08
  in2 : Inport  Port=3  OutDataTypeStr=fixdt(1, 25, 12)  SampleTime=1e-08
  globalSchedule : EnablePort  OutDataTypeStr=boolean
  HwModeRegister : Delay  DelayLength=double(1)  InitialCondition=0
  HwModeRegister1 : Delay  DelayLength=double(1)  InitialCondition=0
  HwModeRegister2 : Delay  DelayLength=double(1)  InitialCondition=0
  PipelineRegister : Delay  DelayLength=double(2)  InitialCondition=0
  _adder_MultiplyAdd : hdlsllib/HDL Operations/Multiply-Add  Function=c+(a.*b)  datatype=fixdt(1, 44, 29)  DoSatur=off  FMA=off
      settings: SourceProductBaseCode=SL
  out0 : Outport  OutDataTypeStr=fixdt(1, 44, 29)  SampleTime=1e-08  InitialOutput=0
  wires:
  PipelineRegister/1 -> out0/1
  in0/1 -> HwModeRegister/1
  in1/1 -> HwModeRegister1/1
  in2/1 -> HwModeRegister2/1
  _adder_MultiplyAdd/1 -> PipelineRegister/1
  HwModeRegister/1 -> _adder_MultiplyAdd/1
  HwModeRegister1/1 -> _adder_MultiplyAdd/2
  HwModeRegister2/1 -> _adder_MultiplyAdd/3

== system gm_uz_pmsm_model_9ph_21b_all_double/uz_pmsm_model_9ph/abc_to_dq/abc_to_dq/_adder_MultiplyAdd38 ==
  in0 : Inport  OutDataTypeStr=fixdt(1, 18, 17)  SampleTime=1e-08
  in1 : Inport  Port=2  OutDataTypeStr=fixdt(1, 25, 12)  SampleTime=1e-08
  in2 : Inport  Port=3  OutDataTypeStr=fixdt(1, 25, 12)  SampleTime=1e-08
  globalSchedule : EnablePort  OutDataTypeStr=boolean
  HwModeRegister : Delay  DelayLength=double(1)  InitialCondition=0
  HwModeRegister1 : Delay  DelayLength=double(1)  InitialCondition=0
  HwModeRegister2 : Delay  DelayLength=double(1)  InitialCondition=0
  PipelineRegister : Delay  DelayLength=double(2)  InitialCondition=0
  _adder_MultiplyAdd : hdlsllib/HDL Operations/Multiply-Add  Function=c+(a.*b)  datatype=fixdt(1, 44, 29)  DoSatur=off  FMA=off
      settings: SourceProductBaseCode=SL
  out0 : Outport  OutDataTypeStr=fixdt(1, 44, 29)  SampleTime=1e-08  InitialOutput=0
  wires:
  PipelineRegister/1 -> out0/1
  in0/1 -> HwModeRegister/1
  in1/1 -> HwModeRegister1/1
  in2/1 -> HwModeRegister2/1
  _adder_MultiplyAdd/1 -> PipelineRegister/1
  HwModeRegister/1 -> _adder_MultiplyAdd/1
  HwModeRegister1/1 -> _adder_MultiplyAdd/2
  HwModeRegister2/1 -> _adder_MultiplyAdd/3

== system gm_uz_pmsm_model_9ph_21b_all_double/uz_pmsm_model_9ph/abc_to_dq/abc_to_dq/_adder_MultiplyAdd39 ==
  in0 : Inport  OutDataTypeStr=fixdt(1, 18, 17)  SampleTime=1e-08
  in1 : Inport  Port=2  OutDataTypeStr=fixdt(1, 25, 12)  SampleTime=1e-08
  in2 : Inport  Port=3  OutDataTypeStr=fixdt(1, 25, 12)  SampleTime=1e-08
  globalSchedule : EnablePort  OutDataTypeStr=boolean
  HwModeRegister : Delay  DelayLength=double(1)  InitialCondition=0
  HwModeRegister1 : Delay  DelayLength=double(1)  InitialCondition=0
  HwModeRegister2 : Delay  DelayLength=double(1)  InitialCondition=0
  PipelineRegister : Delay  DelayLength=double(2)  InitialCondition=0
  _adder_MultiplyAdd : hdlsllib/HDL Operations/Multiply-Add  Function=c+(a.*b)  datatype=fixdt(1, 44, 29)  DoSatur=off  FMA=off
      settings: SourceProductBaseCode=SL
  out0 : Outport  OutDataTypeStr=fixdt(1, 44, 29)  SampleTime=1e-08  InitialOutput=0
  wires:
  PipelineRegister/1 -> out0/1
  in0/1 -> HwModeRegister/1
  in1/1 -> HwModeRegister1/1
  in2/1 -> HwModeRegister2/1
  _adder_MultiplyAdd/1 -> PipelineRegister/1
  HwModeRegister/1 -> _adder_MultiplyAdd/1
  HwModeRegister1/1 -> _adder_MultiplyAdd/2
  HwModeRegister2/1 -> _adder_MultiplyAdd/3

== system gm_uz_pmsm_model_9ph_21b_all_double/uz_pmsm_model_9ph/abc_to_dq/abc_to_dq/_adder_MultiplyAdd4 ==
  in0 : Inport  OutDataTypeStr=fixdt(1, 18, 17)  SampleTime=1e-08
  in1 : Inport  Port=2  OutDataTypeStr=fixdt(1, 25, 12)  SampleTime=1e-08
  in2 : Inport  Port=3  OutDataTypeStr=fixdt(1, 25, 12)  SampleTime=1e-08
  globalSchedule : EnablePort  OutDataTypeStr=boolean
  HwModeRegister : Delay  DelayLength=double(1)  InitialCondition=0
  HwModeRegister1 : Delay  DelayLength=double(1)  InitialCondition=0
  HwModeRegister2 : Delay  DelayLength=double(1)  InitialCondition=0
  PipelineRegister : Delay  DelayLength=double(2)  InitialCondition=0
  _adder_MultiplyAdd : hdlsllib/HDL Operations/Multiply-Add  Function=c+(a.*b)  datatype=fixdt(1, 44, 29)  DoSatur=off  FMA=off
      settings: SourceProductBaseCode=SL
  out0 : Outport  OutDataTypeStr=fixdt(1, 44, 29)  SampleTime=1e-08  InitialOutput=0
  wires:
  PipelineRegister/1 -> out0/1
  in0/1 -> HwModeRegister/1
  in1/1 -> HwModeRegister1/1
  in2/1 -> HwModeRegister2/1
  _adder_MultiplyAdd/1 -> PipelineRegister/1
  HwModeRegister/1 -> _adder_MultiplyAdd/1
  HwModeRegister1/1 -> _adder_MultiplyAdd/2
  HwModeRegister2/1 -> _adder_MultiplyAdd/3

== system gm_uz_pmsm_model_9ph_21b_all_double/uz_pmsm_model_9ph/abc_to_dq/abc_to_dq/_adder_MultiplyAdd40 ==
  in0 : Inport  OutDataTypeStr=fixdt(1, 18, 17)  SampleTime=1e-08
  in1 : Inport  Port=2  OutDataTypeStr=fixdt(1, 25, 12)  SampleTime=1e-08
  in2 : Inport  Port=3  OutDataTypeStr=fixdt(1, 25, 12)  SampleTime=1e-08
  globalSchedule : EnablePort  OutDataTypeStr=boolean
  HwModeRegister : Delay  DelayLength=double(1)  InitialCondition=0
  HwModeRegister1 : Delay  DelayLength=double(1)  InitialCondition=0
  HwModeRegister2 : Delay  DelayLength=double(1)  InitialCondition=0
  PipelineRegister : Delay  DelayLength=double(2)  InitialCondition=0
  _adder_MultiplyAdd : hdlsllib/HDL Operations/Multiply-Add  Function=c+(a.*b)  datatype=fixdt(1, 44, 29)  DoSatur=off  FMA=off
      settings: SourceProductBaseCode=SL
  out0 : Outport  OutDataTypeStr=fixdt(1, 44, 29)  SampleTime=1e-08  InitialOutput=0
  wires:
  PipelineRegister/1 -> out0/1
  in0/1 -> HwModeRegister/1
  in1/1 -> HwModeRegister1/1
  in2/1 -> HwModeRegister2/1
  _adder_MultiplyAdd/1 -> PipelineRegister/1
  HwModeRegister/1 -> _adder_MultiplyAdd/1
  HwModeRegister1/1 -> _adder_MultiplyAdd/2
  HwModeRegister2/1 -> _adder_MultiplyAdd/3

== system gm_uz_pmsm_model_9ph_21b_all_double/uz_pmsm_model_9ph/abc_to_dq/abc_to_dq/_adder_MultiplyAdd41 ==
  in0 : Inport  OutDataTypeStr=fixdt(1, 18, 17)  SampleTime=1e-08
  in1 : Inport  Port=2  OutDataTypeStr=fixdt(1, 25, 12)  SampleTime=1e-08
  in2 : Inport  Port=3  OutDataTypeStr=fixdt(1, 25, 12)  SampleTime=1e-08
  globalSchedule : EnablePort  OutDataTypeStr=boolean
  HwModeRegister : Delay  DelayLength=double(1)  InitialCondition=0
  HwModeRegister1 : Delay  DelayLength=double(1)  InitialCondition=0
  HwModeRegister2 : Delay  DelayLength=double(1)  InitialCondition=0
  PipelineRegister : Delay  DelayLength=double(2)  InitialCondition=0
  _adder_MultiplyAdd : hdlsllib/HDL Operations/Multiply-Add  Function=c+(a.*b)  datatype=fixdt(1, 44, 29)  DoSatur=off  FMA=off
      settings: SourceProductBaseCode=SL
  out0 : Outport  OutDataTypeStr=fixdt(1, 44, 29)  SampleTime=1e-08  InitialOutput=0
  wires:
  PipelineRegister/1 -> out0/1
  in0/1 -> HwModeRegister/1
  in1/1 -> HwModeRegister1/1
  in2/1 -> HwModeRegister2/1
  _adder_MultiplyAdd/1 -> PipelineRegister/1
  HwModeRegister/1 -> _adder_MultiplyAdd/1
  HwModeRegister1/1 -> _adder_MultiplyAdd/2
  HwModeRegister2/1 -> _adder_MultiplyAdd/3

== system gm_uz_pmsm_model_9ph_21b_all_double/uz_pmsm_model_9ph/abc_to_dq/abc_to_dq/_adder_MultiplyAdd42 ==
  in0 : Inport  OutDataTypeStr=fixdt(1, 18, 17)  SampleTime=1e-08
  in1 : Inport  Port=2  OutDataTypeStr=fixdt(1, 25, 12)  SampleTime=1e-08
  in2 : Inport  Port=3  OutDataTypeStr=fixdt(1, 25, 12)  SampleTime=1e-08
  globalSchedule : EnablePort  OutDataTypeStr=boolean
  HwModeRegister : Delay  DelayLength=double(1)  InitialCondition=0
  HwModeRegister1 : Delay  DelayLength=double(1)  InitialCondition=0
  HwModeRegister2 : Delay  DelayLength=double(1)  InitialCondition=0
  PipelineRegister : Delay  DelayLength=double(2)  InitialCondition=0
  _adder_MultiplyAdd : hdlsllib/HDL Operations/Multiply-Add  Function=c+(a.*b)  datatype=fixdt(1, 44, 29)  DoSatur=off  FMA=off
      settings: SourceProductBaseCode=SL
  out0 : Outport  OutDataTypeStr=fixdt(1, 44, 29)  SampleTime=1e-08  InitialOutput=0
  wires:
  PipelineRegister/1 -> out0/1
  in0/1 -> HwModeRegister/1
  in1/1 -> HwModeRegister1/1
  in2/1 -> HwModeRegister2/1
  _adder_MultiplyAdd/1 -> PipelineRegister/1
  HwModeRegister/1 -> _adder_MultiplyAdd/1
  HwModeRegister1/1 -> _adder_MultiplyAdd/2
  HwModeRegister2/1 -> _adder_MultiplyAdd/3

== system gm_uz_pmsm_model_9ph_21b_all_double/uz_pmsm_model_9ph/abc_to_dq/abc_to_dq/_adder_MultiplyAdd43 ==
  in0 : Inport  OutDataTypeStr=fixdt(1, 18, 17)  SampleTime=1e-08
  in1 : Inport  Port=2  OutDataTypeStr=fixdt(1, 25, 12)  SampleTime=1e-08
  in2 : Inport  Port=3  OutDataTypeStr=fixdt(1, 25, 12)  SampleTime=1e-08
  globalSchedule : EnablePort  OutDataTypeStr=boolean
  HwModeRegister : Delay  DelayLength=double(1)  InitialCondition=0
  HwModeRegister1 : Delay  DelayLength=double(1)  InitialCondition=0
  HwModeRegister2 : Delay  DelayLength=double(1)  InitialCondition=0
  PipelineRegister : Delay  DelayLength=double(2)  InitialCondition=0
  _adder_MultiplyAdd : hdlsllib/HDL Operations/Multiply-Add  Function=c+(a.*b)  datatype=fixdt(1, 44, 29)  DoSatur=off  FMA=off
      settings: SourceProductBaseCode=SL
  out0 : Outport  OutDataTypeStr=fixdt(1, 44, 29)  SampleTime=1e-08  InitialOutput=0
  wires:
  PipelineRegister/1 -> out0/1
  in0/1 -> HwModeRegister/1
  in1/1 -> HwModeRegister1/1
  in2/1 -> HwModeRegister2/1
  _adder_MultiplyAdd/1 -> PipelineRegister/1
  HwModeRegister/1 -> _adder_MultiplyAdd/1
  HwModeRegister1/1 -> _adder_MultiplyAdd/2
  HwModeRegister2/1 -> _adder_MultiplyAdd/3

== system gm_uz_pmsm_model_9ph_21b_all_double/uz_pmsm_model_9ph/abc_to_dq/abc_to_dq/_adder_MultiplyAdd44 ==
  in0 : Inport  OutDataTypeStr=fixdt(1, 18, 17)  SampleTime=1e-08
  in1 : Inport  Port=2  OutDataTypeStr=fixdt(1, 25, 12)  SampleTime=1e-08
  in2 : Inport  Port=3  OutDataTypeStr=fixdt(1, 25, 12)  SampleTime=1e-08
  globalSchedule : EnablePort  OutDataTypeStr=boolean
  HwModeRegister : Delay  DelayLength=double(1)  InitialCondition=0
  HwModeRegister1 : Delay  DelayLength=double(1)  InitialCondition=0
  HwModeRegister2 : Delay  DelayLength=double(1)  InitialCondition=0
  PipelineRegister : Delay  DelayLength=double(2)  InitialCondition=0
  _adder_MultiplyAdd : hdlsllib/HDL Operations/Multiply-Add  Function=c+(a.*b)  datatype=fixdt(1, 44, 29)  DoSatur=off  FMA=off
      settings: SourceProductBaseCode=SL
  out0 : Outport  OutDataTypeStr=fixdt(1, 44, 29)  SampleTime=1e-08  InitialOutput=0
  wires:
  PipelineRegister/1 -> out0/1
  in0/1 -> HwModeRegister/1
  in1/1 -> HwModeRegister1/1
  in2/1 -> HwModeRegister2/1
  _adder_MultiplyAdd/1 -> PipelineRegister/1
  HwModeRegister/1 -> _adder_MultiplyAdd/1
  HwModeRegister1/1 -> _adder_MultiplyAdd/2
  HwModeRegister2/1 -> _adder_MultiplyAdd/3

== system gm_uz_pmsm_model_9ph_21b_all_double/uz_pmsm_model_9ph/abc_to_dq/abc_to_dq/_adder_MultiplyAdd45 ==
  in0 : Inport  OutDataTypeStr=fixdt(1, 18, 17)  SampleTime=1e-08
  in1 : Inport  Port=2  OutDataTypeStr=fixdt(1, 25, 12)  SampleTime=1e-08
  in2 : Inport  Port=3  OutDataTypeStr=fixdt(1, 25, 12)  SampleTime=1e-08
  globalSchedule : EnablePort  OutDataTypeStr=boolean
  HwModeRegister : Delay  DelayLength=double(1)  InitialCondition=0
  HwModeRegister1 : Delay  DelayLength=double(1)  InitialCondition=0
  HwModeRegister2 : Delay  DelayLength=double(1)  InitialCondition=0
  PipelineRegister : Delay  DelayLength=double(2)  InitialCondition=0
  _adder_MultiplyAdd : hdlsllib/HDL Operations/Multiply-Add  Function=c+(a.*b)  datatype=fixdt(1, 44, 29)  DoSatur=off  FMA=off
      settings: SourceProductBaseCode=SL
  out0 : Outport  OutDataTypeStr=fixdt(1, 44, 29)  SampleTime=1e-08  InitialOutput=0
  wires:
  PipelineRegister/1 -> out0/1
  in0/1 -> HwModeRegister/1
  in1/1 -> HwModeRegister1/1
  in2/1 -> HwModeRegister2/1
  _adder_MultiplyAdd/1 -> PipelineRegister/1
  HwModeRegister/1 -> _adder_MultiplyAdd/1
  HwModeRegister1/1 -> _adder_MultiplyAdd/2
  HwModeRegister2/1 -> _adder_MultiplyAdd/3

== system gm_uz_pmsm_model_9ph_21b_all_double/uz_pmsm_model_9ph/abc_to_dq/abc_to_dq/_adder_MultiplyAdd46 ==
  in0 : Inport  OutDataTypeStr=fixdt(1, 18, 17)  SampleTime=1e-08
  in1 : Inport  Port=2  OutDataTypeStr=fixdt(1, 25, 12)  SampleTime=1e-08
  in2 : Inport  Port=3  OutDataTypeStr=fixdt(1, 25, 12)  SampleTime=1e-08
  globalSchedule : EnablePort  OutDataTypeStr=boolean
  HwModeRegister : Delay  DelayLength=double(1)  InitialCondition=0
  HwModeRegister1 : Delay  DelayLength=double(1)  InitialCondition=0
  HwModeRegister2 : Delay  DelayLength=double(1)  InitialCondition=0
  PipelineRegister : Delay  DelayLength=double(2)  InitialCondition=0
  _adder_MultiplyAdd : hdlsllib/HDL Operations/Multiply-Add  Function=c+(a.*b)  datatype=fixdt(1, 44, 29)  DoSatur=off  FMA=off
      settings: SourceProductBaseCode=SL
  out0 : Outport  OutDataTypeStr=fixdt(1, 44, 29)  SampleTime=1e-08  InitialOutput=0
  wires:
  PipelineRegister/1 -> out0/1
  in0/1 -> HwModeRegister/1
  in1/1 -> HwModeRegister1/1
  in2/1 -> HwModeRegister2/1
  _adder_MultiplyAdd/1 -> PipelineRegister/1
  HwModeRegister/1 -> _adder_MultiplyAdd/1
  HwModeRegister1/1 -> _adder_MultiplyAdd/2
  HwModeRegister2/1 -> _adder_MultiplyAdd/3

== system gm_uz_pmsm_model_9ph_21b_all_double/uz_pmsm_model_9ph/abc_to_dq/abc_to_dq/_adder_MultiplyAdd47 ==
  in0 : Inport  OutDataTypeStr=fixdt(1, 18, 17)  SampleTime=1e-08
  in1 : Inport  Port=2  OutDataTypeStr=fixdt(1, 25, 12)  SampleTime=1e-08
  in2 : Inport  Port=3  OutDataTypeStr=fixdt(1, 25, 12)  SampleTime=1e-08
  globalSchedule : EnablePort  OutDataTypeStr=boolean
  HwModeRegister : Delay  DelayLength=double(1)  InitialCondition=0
  HwModeRegister1 : Delay  DelayLength=double(1)  InitialCondition=0
  HwModeRegister2 : Delay  DelayLength=double(1)  InitialCondition=0
  PipelineRegister : Delay  DelayLength=double(2)  InitialCondition=0
  _adder_MultiplyAdd : hdlsllib/HDL Operations/Multiply-Add  Function=c+(a.*b)  datatype=fixdt(1, 44, 29)  DoSatur=off  FMA=off
      settings: SourceProductBaseCode=SL
  out0 : Outport  OutDataTypeStr=fixdt(1, 44, 29)  SampleTime=1e-08  InitialOutput=0
  wires:
  PipelineRegister/1 -> out0/1
  in0/1 -> HwModeRegister/1
  in1/1 -> HwModeRegister1/1
  in2/1 -> HwModeRegister2/1
  _adder_MultiplyAdd/1 -> PipelineRegister/1
  HwModeRegister/1 -> _adder_MultiplyAdd/1
  HwModeRegister1/1 -> _adder_MultiplyAdd/2
  HwModeRegister2/1 -> _adder_MultiplyAdd/3

== system gm_uz_pmsm_model_9ph_21b_all_double/uz_pmsm_model_9ph/abc_to_dq/abc_to_dq/_adder_MultiplyAdd48 ==
  in0 : Inport  OutDataTypeStr=fixdt(1, 18, 17)  SampleTime=1e-08
  in1 : Inport  Port=2  OutDataTypeStr=fixdt(1, 25, 12)  SampleTime=1e-08
  in2 : Inport  Port=3  OutDataTypeStr=fixdt(1, 25, 12)  SampleTime=1e-08
  globalSchedule : EnablePort  OutDataTypeStr=boolean
  HwModeRegister : Delay  DelayLength=double(1)  InitialCondition=0
  HwModeRegister1 : Delay  DelayLength=double(1)  InitialCondition=0
  HwModeRegister2 : Delay  DelayLength=double(1)  InitialCondition=0
  PipelineRegister : Delay  DelayLength=double(2)  InitialCondition=0
  _adder_MultiplyAdd : hdlsllib/HDL Operations/Multiply-Add  Function=c+(a.*b)  datatype=fixdt(1, 44, 29)  DoSatur=off  FMA=off
      settings: SourceProductBaseCode=SL
  out0 : Outport  OutDataTypeStr=fixdt(1, 44, 29)  SampleTime=1e-08  InitialOutput=0
  wires:
  PipelineRegister/1 -> out0/1
  in0/1 -> HwModeRegister/1
  in1/1 -> HwModeRegister1/1
  in2/1 -> HwModeRegister2/1
  _adder_MultiplyAdd/1 -> PipelineRegister/1
  HwModeRegister/1 -> _adder_MultiplyAdd/1
  HwModeRegister1/1 -> _adder_MultiplyAdd/2
  HwModeRegister2/1 -> _adder_MultiplyAdd/3
